simulink model "Test_Encoder"  (Simulink 8.1)
settings: Solver=ode45  StartTime=0.0  StopTime=10.0  RelTol=1e-3
libraries: commutil2 x6, Computer_Library x3
settings Model: Creator=N  LastModifiedBy=uzivatel
settings DataIOCC: LimitDataPoints=off  SignalLoggingSaveFormat=Dataset
settings OptimizationCC: ExpressionDepthLimit=128
settings DebuggingCC: UnderspecifiedInitializationDetection=Simplified  MergeDetectMultiDrivingBlocksExec=error  SolverPrmCheckMsg=none  FcnCallInpInsideContextMsg=EnableAllAsError  FrameProcessingCompatibilityMsg=error  StateNameClashWarn=none
settings HardwareCC: ProdBitPerPointer=64  ProdLargestAtomicFloat=Float  ProdIntDivRoundTo=Zero  ProdEndianess=LittleEndian  ProdHWDeviceType=Intel->x86-64 (Windows64)
settings ModelReferenceCC: PropagateSignalLabelsOutOfModel=on
settings GRTTargetCC: CodeReplacementLibrary=None  CombineOutputUpdateFcns=on  CPPClassGenCompliant=on  GRTInterface=off

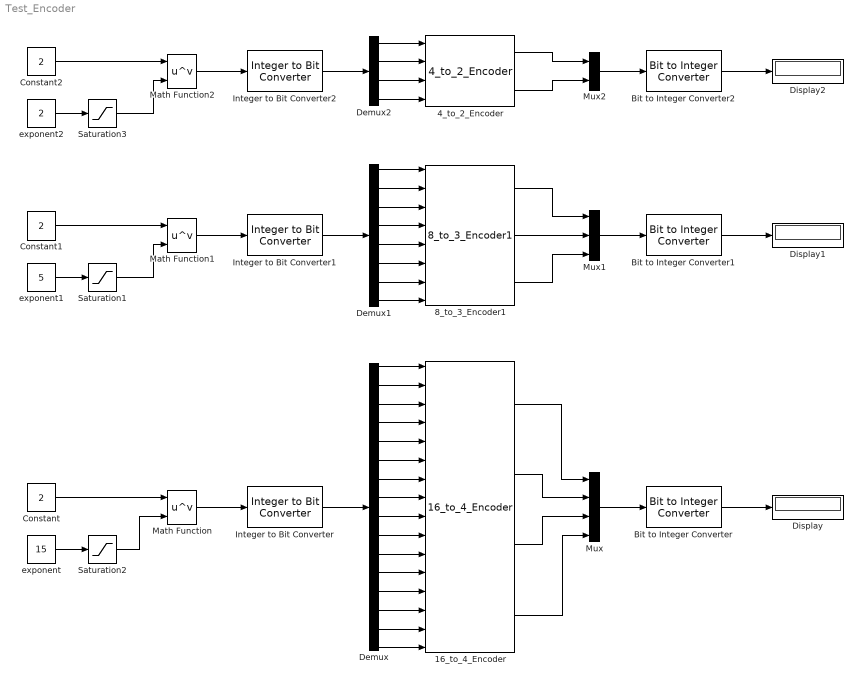
== system Test_Encoder ==
  16_to_4_Encoder : Computer_Library/Encoders/16_to_4_Encoder
  4_to_2_Encoder : Computer_Library/Encoders/4_to_2_Encoder
  8_to_3_Encoder1 : Computer_Library/Encoders/8_to_3_Encoder1
  Bit to Integer Converter : commutil2/Bit to Integer Converter  nbits=4  bitOrder=LSB first  signedOutputValues=Unsigned  outDtype=uint16  outDtypeSigned=Inherit via internal rule
  Bit to Integer Converter1 : commutil2/Bit to Integer Converter  nbits=3  bitOrder=LSB first  signedOutputValues=Unsigned  outDtype=uint16  outDtypeSigned=Inherit via internal rule
  Bit to Integer Converter2 : commutil2/Bit to Integer Converter  nbits=2  bitOrder=LSB first  signedOutputValues=Unsigned  outDtype=uint16  outDtypeSigned=Inherit via internal rule
  Constant : Constant  Value=2
  Constant1 : Constant  Value=2
  Constant2 : Constant  Value=2
  Demux : Demux  Outputs=16
  Demux1 : Demux  Outputs=8
  Demux2 : Demux
  Display : Display
  Display1 : Display
  Display2 : Display
  Integer to Bit Converter : commutil2/Integer to Bit Converter  nbits=16  signedInputValues=Unsigned  bitOrder=LSB first  outDtype=boolean
  Integer to Bit Converter1 : commutil2/Integer to Bit Converter  nbits=8  signedInputValues=Unsigned  bitOrder=LSB first  outDtype=boolean
  Integer to Bit Converter2 : commutil2/Integer to Bit Converter  nbits=4  signedInputValues=Unsigned  bitOrder=LSB first  outDtype=boolean
  Math Function : Math  Operator=pow  SaturateOnIntegerOverflow=on
  Math Function1 : Math  Operator=pow  SaturateOnIntegerOverflow=on
  Math Function2 : Math  Operator=pow  SaturateOnIntegerOverflow=on
  Mux : Mux
  Mux1 : Mux  Inputs=3
  Mux2 : Mux  Inputs=2
  Saturation1 : Saturate  UpperLimit=7  LowerLimit=0
  Saturation2 : Saturate  UpperLimit=15  LowerLimit=0
  Saturation3 : Saturate  UpperLimit=3  LowerLimit=0
  exponent : Constant  Value=15
  exponent1 : Constant  Value=5
  exponent2 : Constant  Value=2
  wires:
  Demux/1 -> 16_to_4_Encoder/1
  Demux/2 -> 16_to_4_Encoder/2
  Demux/3 -> 16_to_4_Encoder/3
  Demux/4 -> 16_to_4_Encoder/4
  Demux/5 -> 16_to_4_Encoder/5
  Demux/7 -> 16_to_4_Encoder/7
  Demux/8 -> 16_to_4_Encoder/8
  Demux/6 -> 16_to_4_Encoder/6
  Demux/9 -> 16_to_4_Encoder/9
  Demux/10 -> 16_to_4_Encoder/10
  Demux/11 -> 16_to_4_Encoder/11
  Demux/12 -> 16_to_4_Encoder/12
  Demux/13 -> 16_to_4_Encoder/13
  Demux/14 -> 16_to_4_Encoder/14
  Demux/15 -> 16_to_4_Encoder/15
  Demux/16 -> 16_to_4_Encoder/16
  16_to_4_Encoder/1 -> Mux/1
  16_to_4_Encoder/4 -> Mux/4
  16_to_4_Encoder/3 -> Mux/3
  16_to_4_Encoder/2 -> Mux/2
  Mux/1 -> Bit to Integer Converter/1
  Bit to Integer Converter/1 -> Display/1
  Integer to Bit Converter/1 -> Demux/1
  Math Function/1 -> Integer to Bit Converter/1
  Constant/1 -> Math Function/1
  Saturation2/1 -> Math Function/2
  exponent/1 -> Saturation2/1
  Integer to Bit Converter1/1 -> Demux1/1
  Math Function1/1 -> Integer to Bit Converter1/1
  Constant1/1 -> Math Function1/1
  Saturation1/1 -> Math Function1/2
  exponent1/1 -> Saturation1/1
  Demux1/1 -> 8_to_3_Encoder1/1
  Demux1/2 -> 8_to_3_Encoder1/2
  Demux1/3 -> 8_to_3_Encoder1/3
  Demux1/4 -> 8_to_3_Encoder1/4
  Demux1/5 -> 8_to_3_Encoder1/5
  Demux1/6 -> 8_to_3_Encoder1/6
  Demux1/7 -> 8_to_3_Encoder1/7
  Demux1/8 -> 8_to_3_Encoder1/8
  Integer to Bit Converter2/1 -> Demux2/1
  Math Function2/1 -> Integer to Bit Converter2/1
  Constant2/1 -> Math Function2/1
  Saturation3/1 -> Math Function2/2
  exponent2/1 -> Saturation3/1
  Demux2/4 -> 4_to_2_Encoder/4
  Demux2/3 -> 4_to_2_Encoder/3
  Demux2/2 -> 4_to_2_Encoder/2
  Demux2/1 -> 4_to_2_Encoder/1
  Mux1/1 -> Bit to Integer Converter1/1
  Bit to Integer Converter1/1 -> Display1/1
  Mux2/1 -> Bit to Integer Converter2/1
  Bit to Integer Converter2/1 -> Display2/1
  8_to_3_Encoder1/2 -> Mux1/2
  8_to_3_Encoder1/1 -> Mux1/1
  8_to_3_Encoder1/3 -> Mux1/3
  4_to_2_Encoder/1 -> Mux2/1
  4_to_2_Encoder/2 -> Mux2/2
